simulink model "trajectory_simulink"  (R2021a)
settings: Solver=ode4  StartTime=0.0  StopTime=10  FixedStep=step_simulation  RelTol=1e-3
values from neighbouring files (symbols this model uses):
  epsilon_sigma = 0.01    [initialization.m]
  k_sigma = k_sigma_best    (= 10)    [initialization.m]
  l_sigma = 5    [initialization.m]
  lambda_sigma = lambda_sigma_best    (= 0.1)    [initialization.m]
undefined symbols (not defined in the file or in its folder): delta_theta_1_2, delta_theta_1_3, delta_theta_2_1, delta_theta_2_3, delta_theta_3_1, delta_theta_3_2, delta_x_1_3, delta_x_2_3, delta_x_3_2, delta_y_1_3, delta_y_2_3, delta_y_3_2
settings Model: Creator=ev_li  LastModifiedBy=mrggi
settings SolverCC: AlgebraicLoopSolver=TrustRegion
settings DebuggingCC: SFMachineParentedDataDiag=warning

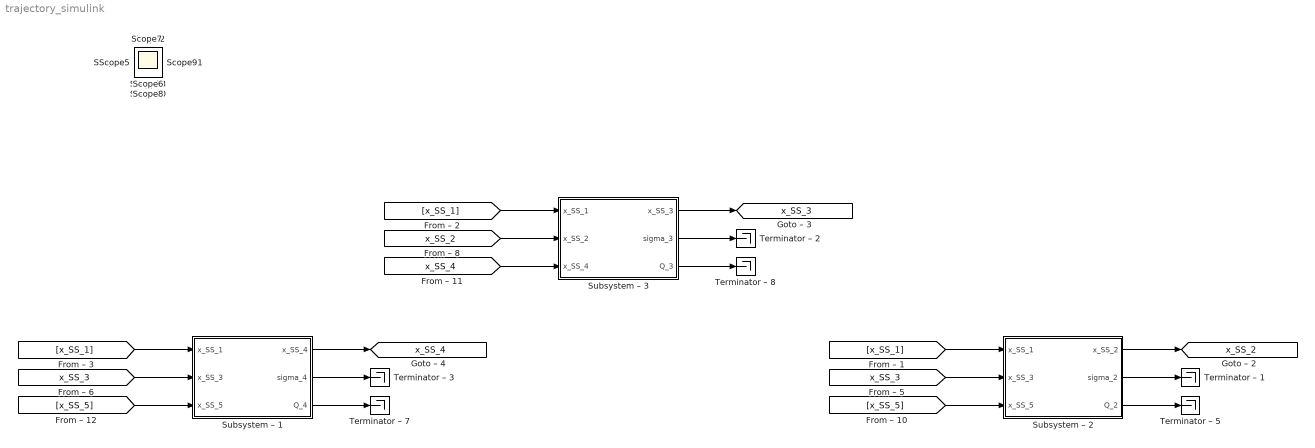
== system trajectory_simulink ==
  Subsystem – 1 : Subsystem
  Subsystem – 2 : Subsystem
  Subsystem – 3 : Subsystem
  Terminator – {1..3,5,7..8} (6 alike) : Terminator
  Scope{,1..13} (14 alike) : Scope
  tag scope: x_SS_2=global, x_SS_3=global, x_SS_4=global
  wires:
  Subsystem – 2/1(x_SS_2) -> [x_SS_2]
  Subsystem – 3/1(x_SS_3) -> [x_SS_3]
  Subsystem – 1/1(x_SS_4) -> [x_SS_4]
  [x_SS_1] -> Subsystem – 2/1(x_SS_1)
  [x_SS_1] -> Subsystem – 3/1(x_SS_1)
  [x_SS_1] -> Subsystem – 1/1(x_SS_1)
  [x_SS_3] -> Subsystem – 2/2(x_SS_3)
  [x_SS_3] -> Subsystem – 1/2(x_SS_3)
  [x_SS_2] -> Subsystem – 3/2(x_SS_2)
  [x_SS_5] -> Subsystem – 2/3(x_SS_5)
  [x_SS_4] -> Subsystem – 3/3(x_SS_4)
  [x_SS_5] -> Subsystem – 1/3(x_SS_5)
  Subsystem – 2/2(sigma_2) -> Terminator – 1/1
  Subsystem – 3/2(sigma_3) -> Terminator – 2/1
  Subsystem – 1/2(sigma_4) -> Terminator – 3/1
  Subsystem – 2/3(Q_2) -> Terminator – 5/1
  Subsystem – 1/3(Q_4) -> Terminator – 7/1
  Subsystem – 3/3(Q_3) -> Terminator – 8/1

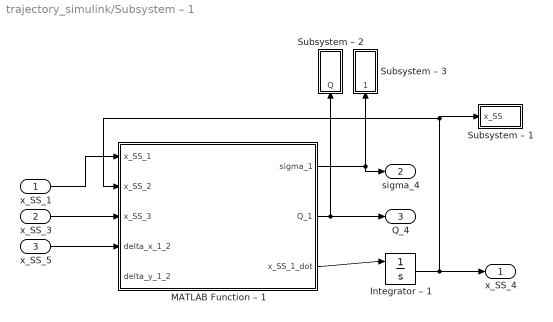
== system trajectory_simulink/Subsystem – 1 ==
  x_SS_1 : Inport
  x_SS_3 : Inport  Port=2
  x_SS_5 : Inport  Port=3
  Integrator – 1 : Integrator  InitialConditionSource=external
  MATLAB Function – 1 : MATLAB Function  TreatAsAtomicUnit=on
  Subsystem – 1 : Subsystem
  Subsystem – 2 : Subsystem
  Subsystem – 3 : Subsystem
  x_SS_4 : Outport
  sigma_4 : Outport  Port=2
  Q_4 : Outport  Port=3
  wires:
  MATLAB Function – 1/3(x_SS_1_dot) -> Integrator – 1/1
  x_SS_1/1 -> MATLAB Function – 1/1(x_SS_1)
  x_SS_3/1 -> MATLAB Function – 1/3(x_SS_3)
  x_SS_5/1 -> MATLAB Function – 1/4(delta_x_1_2)
  MATLAB Function – 1/1(sigma_1) -> Subsystem – 3/1(sigma), sigma_4/1
  MATLAB Function – 1/2(Q_1) -> Subsystem – 2/1(Q), Q_4/1
  Integrator – 1/1 -> Subsystem – 1/1(x_SS), MATLAB Function – 1/2(x_SS_2), x_SS_4/1

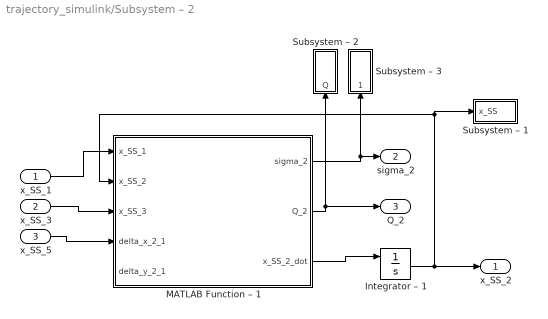
== system trajectory_simulink/Subsystem – 2 ==
  x_SS_1 : Inport
  x_SS_3 : Inport  Port=2
  x_SS_5 : Inport  Port=3
  Integrator – 1 : Integrator  InitialConditionSource=external
  MATLAB Function – 1 : MATLAB Function  TreatAsAtomicUnit=on
  Subsystem – 1 : Subsystem
  Subsystem – 2 : Subsystem
  Subsystem – 3 : Subsystem
  x_SS_2 : Outport
  sigma_2 : Outport  Port=2
  Q_2 : Outport  Port=3
  wires:
  MATLAB Function – 1/3(x_SS_2_dot) -> Integrator – 1/1
  x_SS_3/1 -> MATLAB Function – 1/3(x_SS_3)
  x_SS_5/1 -> MATLAB Function – 1/4(delta_x_2_1)
  x_SS_1/1 -> MATLAB Function – 1/1(x_SS_1)
  MATLAB Function – 1/1(sigma_2) -> sigma_2/1, Subsystem – 3/1(sigma)
  MATLAB Function – 1/2(Q_2) -> Subsystem – 2/1(Q), Q_2/1
  Integrator – 1/1 -> Subsystem – 1/1(x_SS), MATLAB Function – 1/2(x_SS_2), x_SS_2/1

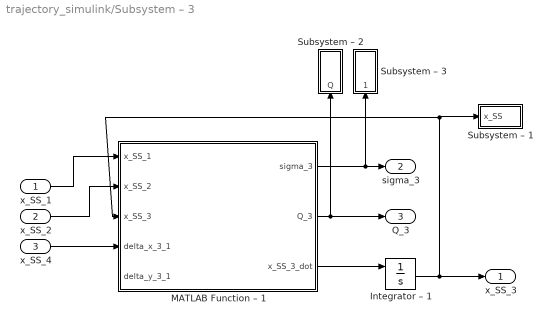
== system trajectory_simulink/Subsystem – 3 ==
  x_SS_1 : Inport
  x_SS_2 : Inport  Port=2
  x_SS_4 : Inport  Port=3
  Integrator – 1 : Integrator  InitialConditionSource=external
  MATLAB Function – 1 : MATLAB Function  TreatAsAtomicUnit=on
  Subsystem – 1 : Subsystem
  Subsystem – 2 : Subsystem
  Subsystem – 3 : Subsystem
  x_SS_3 : Outport
  sigma_3 : Outport  Port=2
  Q_3 : Outport  Port=3
  wires:
  MATLAB Function – 1/3(x_SS_3_dot) -> Integrator – 1/1
  x_SS_2/1 -> MATLAB Function – 1/2(x_SS_2)
  x_SS_4/1 -> MATLAB Function – 1/4(delta_x_3_1)
  x_SS_1/1 -> MATLAB Function – 1/1(x_SS_1)
  MATLAB Function – 1/1(sigma_3) -> Subsystem – 3/1(sigma), sigma_3/1
  MATLAB Function – 1/2(Q_3) -> Subsystem – 2/1(Q), Q_3/1
  Integrator – 1/1 -> Subsystem – 1/1(x_SS), MATLAB Function – 1/3(x_SS_3), x_SS_3/1

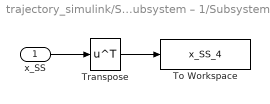
== system trajectory_simulink/Subsystem – 1/Subsystem – 1 ==
  x_SS : Inport
  To Workspace : ToWorkspace  VariableName=x_SS_4  SampleTime=-1
      settings: Save2DSignal=2-D array (concatenate along first dimension)
  Transpose : Math  Operator=transpose  SaturateOnIntegerOverflow=on
  wires:
  Transpose/1 -> To Workspace/1
  x_SS/1 -> Transpose/1

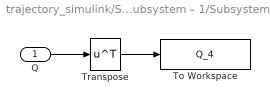
== system trajectory_simulink/Subsystem – 1/Subsystem – 2 ==
  Q : Inport
  To Workspace : ToWorkspace  VariableName=Q_4  SampleTime=-1
      settings: Save2DSignal=2-D array (concatenate along first dimension)
  Transpose : Math  Operator=transpose  SaturateOnIntegerOverflow=on
  wires:
  Transpose/1 -> To Workspace/1
  Q/1 -> Transpose/1

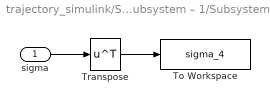
== system trajectory_simulink/Subsystem – 1/Subsystem – 3 ==
  sigma : Inport
  To Workspace : ToWorkspace  VariableName=sigma_4  SampleTime=-1
      settings: Save2DSignal=2-D array (concatenate along first dimension)
  Transpose : Math  Operator=transpose  SaturateOnIntegerOverflow=on
  wires:
  Transpose/1 -> To Workspace/1
  sigma/1 -> Transpose/1

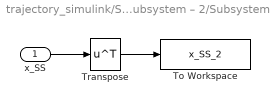
== system trajectory_simulink/Subsystem – 2/Subsystem – 1 ==
  x_SS : Inport
  To Workspace : ToWorkspace  VariableName=x_SS_2  SampleTime=-1
      settings: Save2DSignal=2-D array (concatenate along first dimension)
  Transpose : Math  Operator=transpose  SaturateOnIntegerOverflow=on
  wires:
  Transpose/1 -> To Workspace/1
  x_SS/1 -> Transpose/1

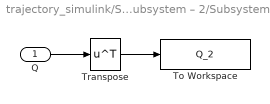
== system trajectory_simulink/Subsystem – 2/Subsystem – 2 ==
  Q : Inport
  To Workspace : ToWorkspace  VariableName=Q_2  SampleTime=-1
      settings: Save2DSignal=2-D array (concatenate along first dimension)
  Transpose : Math  Operator=transpose  SaturateOnIntegerOverflow=on
  wires:
  Transpose/1 -> To Workspace/1
  Q/1 -> Transpose/1

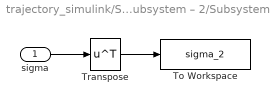
== system trajectory_simulink/Subsystem – 2/Subsystem – 3 ==
  sigma : Inport
  To Workspace : ToWorkspace  VariableName=sigma_2  SampleTime=-1
      settings: Save2DSignal=2-D array (concatenate along first dimension)
  Transpose : Math  Operator=transpose  SaturateOnIntegerOverflow=on
  wires:
  Transpose/1 -> To Workspace/1
  sigma/1 -> Transpose/1

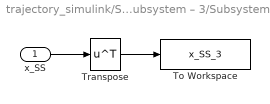
== system trajectory_simulink/Subsystem – 3/Subsystem – 1 ==
  x_SS : Inport
  To Workspace : ToWorkspace  VariableName=x_SS_3  SampleTime=-1
      settings: Save2DSignal=2-D array (concatenate along first dimension)
  Transpose : Math  Operator=transpose  SaturateOnIntegerOverflow=on
  wires:
  Transpose/1 -> To Workspace/1
  x_SS/1 -> Transpose/1

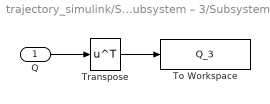
== system trajectory_simulink/Subsystem – 3/Subsystem – 2 ==
  Q : Inport
  To Workspace : ToWorkspace  VariableName=Q_3  SampleTime=-1
      settings: Save2DSignal=2-D array (concatenate along first dimension)
  Transpose : Math  Operator=transpose  SaturateOnIntegerOverflow=on
  wires:
  Transpose/1 -> To Workspace/1
  Q/1 -> Transpose/1

== system trajectory_simulink/Subsystem – 3/Subsystem – 3 ==
  sigma : Inport
  To Workspace : ToWorkspace  VariableName=sigma_3  SampleTime=-1
      settings: Save2DSignal=2-D array (concatenate along first dimension)
  Transpose : Math  Operator=transpose  SaturateOnIntegerOverflow=on
  wires:
  Transpose/1 -> To Workspace/1
  sigma/1 -> Transpose/1

== matlab function trajectory_simulink/Subsystem – 1/MATLAB Function – 1 ==
  data: x_SS_1 input; sigma_1 output; Q_1 output; x_SS_2 input; x_SS_3 input; lambda_sigma parameter; k_sigma parameter; l_sigma parameter; epsilon_sigma parameter; delta_x_1_2 input; delta_y_1_2 input; x_SS_1_dot output; delta_theta_1_2 parameter; delta_x_1_3 parameter; delta_y_1_3 parameter; delta_theta_1_3 parameter
function [sigma_1,Q_1,x_SS_1_dot]=fcn(x_SS_1,x_SS_2,x_SS_3,...
    lambda_sigma,k_sigma,l_sigma,epsilon_sigma,...
    delta_x_1_2,delta_y_1_2,delta_theta_1_2,...
    delta_x_1_3,delta_y_1_3,delta_theta_1_3)

%% INPUTS

x_1=x_SS_1(1);
y_1=x_SS_1(2);
theta_1=x_SS_1(3);

u_1=x_SS_1(4);
v_1=x_SS_1(5);
r_1=x_SS_1(6);

x_1=x_SS_1(1);
y_1=x_SS_1(2);
theta_1=x_SS_1(3);

u_1=x_SS_1(4);
v_1=x_SS_1(5);
r_1=x_SS_1(6);

u_1_dot=0;
v_1_dot=0;
r_1_dot=0;

x_2=x_SS_2(1);
y_2=x_SS_2(2);
theta_2=x_SS_2(3);

u_2=x_SS_2(4);
v_2=x_SS_2(5);
r_2=x_SS_2(6);

u_2_dot=0;
v_2_dot=0;
r_2_dot=0;

x_3=x_SS_3(1);
y_3=x_SS_3(2);
theta_3=x_SS_3(3);

u_3=x_SS_3(4);
v_3=x_SS_3(5);
r_3=x_SS_3(6);

u_3_dot=0;
v_3_dot=0;
r_3_dot=0;

%% FORMATION

A_c=[[ 2*cos(theta_3), 2*sin(theta_3), 0];
     [-2*sin(theta_3), 2*cos(theta_3), 0];
     [              0,              0, 2];];

b_c=[k_sigma*tanh((lambda_sigma*(delta_x_1_2+x_2)+lambda_sigma*(delta_x_1_3+x_3)-2*lambda_sigma*x_1-2*u_1*cos(theta_1)+u_2*cos(theta_2)+u_3*cos(theta_3)-2*v_1*sin(theta_1)+v_2*sin(theta_2)+v_3*sin(theta_3))/epsilon_sigma)-2*lambda_sigma*(u_1*cos(theta_1)+v_1*sin(theta_1))+lambda_sigma*(u_2*cos(theta_2)+v_2*sin(theta_2))+lambda_sigma*(u_3*cos(theta_3)+v_3*sin(theta_3))+u_2_dot*cos(theta_2)+u_3_dot*cos(theta_3)+v_2_dot*sin(theta_2)+v_3_dot*sin(theta_3)+l_sigma*(lambda_sigma*(delta_x_1_2+x_2)+lambda_sigma*(delta_x_1_3+x_3)-2*lambda_sigma*x_1-2*u_1*cos(theta_1)+u_2*cos(theta_2)+u_3*cos(theta_3)-2*v_1*sin(theta_1)+v_2*sin(theta_2)+v_3*sin(theta_3))-2*r_1*v_1*cos(theta_1)+r_2*v_2*cos(theta_2)+r_3*v_3*cos(theta_3)+2*r_1*u_1*sin(theta_1)-r_2*u_2*sin(theta_2)-r_3*u_3*sin(theta_3);
k_sigma*tanh((lambda_sigma*(delta_y_1_2+y_2)+lambda_sigma*(delta_y_1_3+y_3)-2*lambda_sigma*y_1-2*v_1*cos(theta_1)+v_2*cos(theta_2)+v_3*cos(theta_3)+2*u_1*sin(theta_1)-u_2*sin(theta_2)-u_3*sin(theta_3))/epsilon_sigma)-2*lambda_sigma*(v_1*cos(theta_1)-u_1*sin(theta_1))+lambda_sigma*(v_2*cos(theta_2)-u_2*sin(theta_2))+lambda_sigma*(v_3*cos(theta_3)-u_3*sin(theta_3))+v_2_dot*cos(theta_2)+v_3_dot*cos(theta_3)-u_2_dot*sin(theta_2)-u_3_dot*sin(theta_3)+l_sigma*(lambda_sigma*(delta_y_1_2+y_2)+lambda_sigma*(delta_y_1_3+y_3)-2*lambda_sigma*y_1-2*v_1*cos(theta_1)+v_2*cos(theta_2)+v_3*cos(theta_3)+2*u_1*sin(theta_1)-u_2*sin(theta_2)-u_3*sin(theta_3))+2*r_1*u_1*cos(theta_1)-r_2*u_2*cos(theta_2)-r_3*u_3*cos(theta_3)+2*r_1*v_1*sin(theta_1)-r_2*v_2*sin(theta_2)-r_3*v_3*sin(theta_3);
r_2_dot+r_3_dot+l_sigma*(r_2-2*r_1+r_3+lambda_sigma*(delta_theta_1_2+theta_2)+lambda_sigma*(delta_theta_1_3+theta_3)-2*lambda_sigma*theta_1)-2*lambda_sigma*r_1+lambda_sigma*r_2+lambda_sigma*r_3+k_sigma*tanh((r_2-2*r_1+r_3+lambda_sigma*(delta_theta_1_2+theta_2)+lambda_sigma*(delta_theta_1_3+theta_3)-2*lambda_sigma*theta_1)/epsilon_sigma);];

sigma_1=[2*lambda_sigma*x_1 - lambda_sigma*(delta_x_1_3 + x_3) - lambda_sigma*(delta_x_1_2 + x_2) + 2*u_1*cos(theta_1) - u_2*cos(theta_2) - u_3*cos(theta_3) + 2*v_1*sin(theta_1) - v_2*sin(theta_2) - v_3*sin(theta_3);
2*lambda_sigma*y_1 - lambda_sigma*(delta_y_1_3 + y_3) - lambda_sigma*(delta_y_1_2 + y_2) + 2*v_1*cos(theta_1) - v_2*cos(theta_2) - v_3*cos(theta_3) - 2*u_1*sin(theta_1) + u_2*sin(theta_2) + u_3*sin(theta_3);
2*r_1-r_2-r_3-lambda_sigma*(delta_theta_1_2+theta_2)-lambda_sigma*(delta_theta_1_3+theta_3)+2*lambda_sigma*theta_1;];


%% REFERENCE MODEL

[nu,R,M,tau]=UGV_dynamics(x_1,y_1,theta_1,u_1,v_1,r_1);

%% TRAJECTORY GENERATOR

[x_SS_1_dot,Q_1]=cooperative_filter(A_c,b_c,nu,R,M,tau);

end

== matlab function trajectory_simulink/Subsystem – 3/MATLAB Function – 1 ==
  data: x_SS_1 input; x_SS_2 input; sigma_3 output; Q_3 output; x_SS_3 input; lambda_sigma parameter; k_sigma parameter; l_sigma parameter; epsilon_sigma parameter; delta_x_3_1 input; delta_y_3_1 input; x_SS_3_dot output; delta_theta_3_1 parameter; delta_x_3_2 parameter; delta_y_3_2 parameter; delta_theta_3_2 parameter
function [sigma_3,Q_3,x_SS_3_dot]=fcn(x_SS_1,x_SS_2,x_SS_3,...
    lambda_sigma,k_sigma,l_sigma,epsilon_sigma,...
    delta_x_3_1,delta_y_3_1,delta_theta_3_1,...
    delta_x_3_2,delta_y_3_2,delta_theta_3_2)

%% INPUTS

x_1=x_SS_1(1);
y_1=x_SS_1(2);
theta_1=x_SS_1(3);

u_1=x_SS_1(4);
v_1=x_SS_1(5);
r_1=x_SS_1(6);

x_1=x_SS_1(1);
y_1=x_SS_1(2);
theta_1=x_SS_1(3);

u_1=x_SS_1(4);
v_1=x_SS_1(5);
r_1=x_SS_1(6);

u_1_dot=0;
v_1_dot=0;
r_1_dot=0;

x_2=x_SS_2(1);
y_2=x_SS_2(2);
theta_2=x_SS_2(3);

u_2=x_SS_2(4);
v_2=x_SS_2(5);
r_2=x_SS_2(6);

u_2_dot=0;
v_2_dot=0;
r_2_dot=0;

x_3=x_SS_3(1);
y_3=x_SS_3(2);
theta_3=x_SS_3(3);

u_3=x_SS_3(4);
v_3=x_SS_3(5);
r_3=x_SS_3(6);

u_3_dot=0;
v_3_dot=0;
r_3_dot=0;

%% FORMATION

A_c=[[ 2*cos(theta_3), 2*sin(theta_3), 0];
     [-2*sin(theta_3), 2*cos(theta_3), 0];
     [              0,              0, 2];];

b_c=[k_sigma*tanh((lambda_sigma*(delta_x_3_1 + x_1) + lambda_sigma*(delta_x_3_2 + x_2) - 2*lambda_sigma*x_3 + u_1*cos(theta_1) + u_2*cos(theta_2) - 2*u_3*cos(theta_3) + v_1*sin(theta_1) + v_2*sin(theta_2) - 2*v_3*sin(theta_3))/epsilon_sigma) + lambda_sigma*(u_1*cos(theta_1) + v_1*sin(theta_1)) + lambda_sigma*(u_2*cos(theta_2) + v_2*sin(theta_2)) - 2*lambda_sigma*(u_3*cos(theta_3) + v_3*sin(theta_3)) + u_1_dot*cos(theta_1) + u_2_dot*cos(theta_2) + v_1_dot*sin(theta_1) + v_2_dot*sin(theta_2) + l_sigma*(lambda_sigma*(delta_x_3_1 + x_1) + lambda_sigma*(delta_x_3_2 + x_2) - 2*lambda_sigma*x_3 + u_1*cos(theta_1) + u_2*cos(theta_2) - 2*u_3*cos(theta_3) + v_1*sin(theta_1) + v_2*sin(theta_2) - 2*v_3*sin(theta_3)) + r_1*v_1*cos(theta_1) + r_2*v_2*cos(theta_2) - 2*r_3*v_3*cos(theta_3) - r_1*u_1*sin(theta_1) - r_2*u_2*sin(theta_2) + 2*r_3*u_3*sin(theta_3);
k_sigma*tanh((lambda_sigma*(delta_y_3_1 + y_1) + lambda_sigma*(delta_y_3_2 + y_2) - 2*lambda_sigma*y_3 + v_1*cos(theta_1) + v_2*cos(theta_2) - 2*v_3*cos(theta_3) - u_1*sin(theta_1) - u_2*sin(theta_2) + 2*u_3*sin(theta_3))/epsilon_sigma) + lambda_sigma*(v_1*cos(theta_1) - u_1*sin(theta_1)) + lambda_sigma*(v_2*cos(theta_2) - u_2*sin(theta_2)) - 2*lambda_sigma*(v_3*cos(theta_3) - u_3*sin(theta_3)) + v_1_dot*cos(theta_1) + v_2_dot*cos(theta_2) - u_1_dot*sin(theta_1) - u_2_dot*sin(theta_2) + l_sigma*(lambda_sigma*(delta_y_3_1 + y_1) + lambda_sigma*(delta_y_3_2 + y_2) - 2*lambda_sigma*y_3 + v_1*cos(theta_1) + v_2*cos(theta_2) - 2*v_3*cos(theta_3) - u_1*sin(theta_1) - u_2*sin(theta_2) + 2*u_3*sin(theta_3)) - r_1*u_1*cos(theta_1) - r_2*u_2*cos(theta_2) + 2*r_3*u_3*cos(theta_3) - r_1*v_1*sin(theta_1) - r_2*v_2*sin(theta_2) + 2*r_3*v_3*sin(theta_3);
r_1_dot+r_2_dot+l_sigma*(r_1+r_2-2*r_3+lambda_sigma*(delta_theta_3_1+theta_1)+lambda_sigma*(delta_theta_3_2+theta_2)-2*lambda_sigma*theta_3)+lambda_sigma*r_1+lambda_sigma*r_2-2*lambda_sigma*r_3+k_sigma*tanh((r_1+r_2-2*r_3+lambda_sigma*(delta_theta_3_1+theta_1)+lambda_sigma*(delta_theta_3_2+theta_2)-2*lambda_sigma*theta_3)/epsilon_sigma);];

sigma_3=[2*lambda_sigma*x_3 - lambda_sigma*(delta_x_3_2 + x_2) - lambda_sigma*(delta_x_3_1 + x_1) - u_1*cos(theta_1) - u_2*cos(theta_2) + 2*u_3*cos(theta_3) - v_1*sin(theta_1) - v_2*sin(theta_2) + 2*v_3*sin(theta_3);
2*lambda_sigma*y_3 - lambda_sigma*(delta_y_3_2 + y_2) - lambda_sigma*(delta_y_3_1 + y_1) - v_1*cos(theta_1) - v_2*cos(theta_2) + 2*v_3*cos(theta_3) + u_1*sin(theta_1) + u_2*sin(theta_2) - 2*u_3*sin(theta_3);
2*r_3-r_2-r_1-lambda_sigma*(delta_theta_3_1+theta_1)-lambda_sigma*(delta_theta_3_2+theta_2)+2*lambda_sigma*theta_3;];

%% REFERENCE MODEL

[nu,R,M,tau]=UGV_dynamics(x_3,y_3,theta_3,u_3,v_3,r_3);

%% TRAJECTORY GENERATOR

[x_SS_3_dot,Q_3]=cooperative_filter(A_c,b_c,nu,R,M,tau);

end

== matlab function trajectory_simulink/Subsystem – 2/MATLAB Function – 1 ==
  data: x_SS_1 input; sigma_2 output; Q_2 output; x_SS_2 input; x_SS_3 input; lambda_sigma parameter; k_sigma parameter; l_sigma parameter; epsilon_sigma parameter; delta_x_2_1 input; delta_y_2_1 input; x_SS_2_dot output; delta_theta_2_1 parameter; delta_x_2_3 parameter; delta_y_2_3 parameter; delta_theta_2_3 parameter
function [sigma_2,Q_2,x_SS_2_dot]=fcn(x_SS_1,x_SS_2,x_SS_3,...
    lambda_sigma,k_sigma,l_sigma,epsilon_sigma,...
    delta_x_2_1,delta_y_2_1,delta_theta_2_1,...
    delta_x_2_3,delta_y_2_3,delta_theta_2_3)

%% INPUTS

x_1=x_SS_1(1);
y_1=x_SS_1(2);
theta_1=x_SS_1(3);

u_1=x_SS_1(4);
v_1=x_SS_1(5);
r_1=x_SS_1(6);

x_1=x_SS_1(1);
y_1=x_SS_1(2);
theta_1=x_SS_1(3);

u_1=x_SS_1(4);
v_1=x_SS_1(5);
r_1=x_SS_1(6);

u_1_dot=0;
v_1_dot=0;
r_1_dot=0;

x_2=x_SS_2(1);
y_2=x_SS_2(2);
theta_2=x_SS_2(3);

u_2=x_SS_2(4);
v_2=x_SS_2(5);
r_2=x_SS_2(6);

u_2_dot=0;
v_2_dot=0;
r_2_dot=0;

x_3=x_SS_3(1);
y_3=x_SS_3(2);
theta_3=x_SS_3(3);

u_3=x_SS_3(4);
v_3=x_SS_3(5);
r_3=x_SS_3(6);

u_3_dot=0;
v_3_dot=0;
r_3_dot=0;

%% FORMATION

A_c=[[ 2*cos(theta_3), 2*sin(theta_3), 0];
     [-2*sin(theta_3), 2*cos(theta_3), 0];
     [              0,              0, 2];];

b_c=[k_sigma*tanh((lambda_sigma*(delta_x_2_1 + x_1) + lambda_sigma*(delta_x_2_3 + x_3) - 2*lambda_sigma*x_2 + u_1*cos(theta_1) - 2*u_2*cos(theta_2) + u_3*cos(theta_3) + v_1*sin(theta_1) - 2*v_2*sin(theta_2) + v_3*sin(theta_3))/epsilon_sigma) + lambda_sigma*(u_1*cos(theta_1) + v_1*sin(theta_1)) - 2*lambda_sigma*(u_2*cos(theta_2) + v_2*sin(theta_2)) + lambda_sigma*(u_3*cos(theta_3) + v_3*sin(theta_3)) + u_1_dot*cos(theta_1) + u_3_dot*cos(theta_3) + v_1_dot*sin(theta_1) + v_3_dot*sin(theta_3) + l_sigma*(lambda_sigma*(delta_x_2_1 + x_1) + lambda_sigma*(delta_x_2_3 + x_3) - 2*lambda_sigma*x_2 + u_1*cos(theta_1) - 2*u_2*cos(theta_2) + u_3*cos(theta_3) + v_1*sin(theta_1) - 2*v_2*sin(theta_2) + v_3*sin(theta_3)) + r_1*v_1*cos(theta_1) - 2*r_2*v_2*cos(theta_2) + r_3*v_3*cos(theta_3) - r_1*u_1*sin(theta_1) + 2*r_2*u_2*sin(theta_2) - r_3*u_3*sin(theta_3);
k_sigma*tanh((lambda_sigma*(delta_y_2_1 + y_1) + lambda_sigma*(delta_y_2_3 + y_3) - 2*lambda_sigma*y_2 + v_1*cos(theta_1) - 2*v_2*cos(theta_2) + v_3*cos(theta_3) - u_1*sin(theta_1) + 2*u_2*sin(theta_2) - u_3*sin(theta_3))/epsilon_sigma) + lambda_sigma*(v_1*cos(theta_1) - u_1*sin(theta_1)) - 2*lambda_sigma*(v_2*cos(theta_2) - u_2*sin(theta_2)) + lambda_sigma*(v_3*cos(theta_3) - u_3*sin(theta_3)) + v_1_dot*cos(theta_1) + v_3_dot*cos(theta_3) - u_1_dot*sin(theta_1) - u_3_dot*sin(theta_3) + l_sigma*(lambda_sigma*(delta_y_2_1 + y_1) + lambda_sigma*(delta_y_2_3 + y_3) - 2*lambda_sigma*y_2 + v_1*cos(theta_1) - 2*v_2*cos(theta_2) + v_3*cos(theta_3) - u_1*sin(theta_1) + 2*u_2*sin(theta_2) - u_3*sin(theta_3)) - r_1*u_1*cos(theta_1) + 2*r_2*u_2*cos(theta_2) - r_3*u_3*cos(theta_3) - r_1*v_1*sin(theta_1) + 2*r_2*v_2*sin(theta_2) - r_3*v_3*sin(theta_3);
r_1_dot+r_3_dot+l_sigma*(r_1-2*r_2+r_3+lambda_sigma*(delta_theta_2_1+theta_1)+lambda_sigma*(delta_theta_2_3+theta_3)-2*lambda_sigma*theta_2)+lambda_sigma*r_1-2*lambda_sigma*r_2+lambda_sigma*r_3+k_sigma*tanh((r_1-2*r_2+r_3+lambda_sigma*(delta_theta_2_1+theta_1)+lambda_sigma*(delta_theta_2_3+theta_3)-2*lambda_sigma*theta_2)/epsilon_sigma);];

sigma_2=[2*lambda_sigma*x_2 - lambda_sigma*(delta_x_2_3 + x_3) - lambda_sigma*(delta_x_2_1 + x_1) - u_1*cos(theta_1) + 2*u_2*cos(theta_2) - u_3*cos(theta_3) - v_1*sin(theta_1) + 2*v_2*sin(theta_2) - v_3*sin(theta_3);
2*lambda_sigma*y_2 - lambda_sigma*(delta_y_2_3 + y_3) - lambda_sigma*(delta_y_2_1 + y_1) - v_1*cos(theta_1) + 2*v_2*cos(theta_2) - v_3*cos(theta_3) + u_1*sin(theta_1) - 2*u_2*sin(theta_2) + u_3*sin(theta_3);
2*r_2-r_1-r_3-lambda_sigma*(delta_theta_2_1+theta_1)-lambda_sigma*(delta_theta_2_3+theta_3)+2*lambda_sigma*theta_2;];


%% REFERENCE MODEL

[nu,R,M,tau]=UGV_dynamics(x_2,y_2,theta_2,u_2,v_2,r_2);

%% TRAJECTORY GENERATOR

[x_SS_2_dot,Q_2]=cooperative_filter(A_c,b_c,nu,R,M,tau);

end
